simulink model "cp"  (R2012b)
settings: Solver=FixedStepDiscrete  SolverMode=SingleTasking  StartTime=0.0  StopTime=5000  RelTol=1e-3
libraries: shlslibv1 x19
settings Model: synDspstartup=OK  Creator=sszilvasi  LastModifiedBy=sszilvasi
settings DataIOCC: SaveOutput=off  SignalLogging=off  SaveTime=off
settings OptimizationCC: InlineParams=on
settings DebuggingCC: AlgebraicLoopMsg=error  InheritedTsInSrcMsg=none

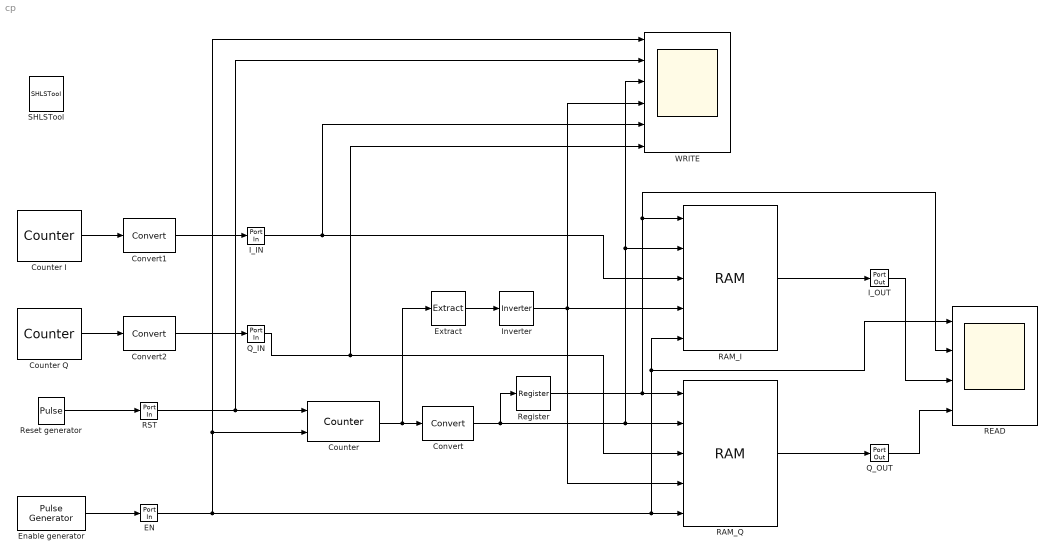
== system cp ==
  Convert : shlslibv1/Signal Operations/Convert  syn_preshift_opr=none  syn_preshift_bits=0  syn_preshift_val=0  syn_out_f=Specify  syn_out_wl=5  syn_out_fl=0  syn_out_dt_sync=unsigned  syn_out_sat=off  syn_out_rnd=Floor (Truncate)  syn_inh_port=off  syn_inh_st=off  syn_inh_stf=1  synBlockType=primitive  synLatency=0  synBlockId=4
  Convert1 : shlslibv1/Signal Operations/Convert  syn_preshift_opr=>>  syn_preshift_bits=9  syn_preshift_val=0  syn_out_f=Specify  syn_out_wl=10  syn_out_fl=9  syn_out_dt_sync=signed  syn_out_sat=off  syn_out_rnd=Floor (Truncate)  syn_inh_port=off  syn_inh_st=off  syn_inh_stf=1  synBlockType=primitive  synLatency=0  synBlockId=4
  Convert2 : shlslibv1/Signal Operations/Convert  syn_preshift_opr=>>  syn_preshift_bits=9  syn_preshift_val=0  syn_out_f=Specify  syn_out_wl=10  syn_out_fl=9  syn_out_dt_sync=signed  syn_out_sat=off  syn_out_rnd=Floor (Truncate)  syn_inh_port=off  syn_inh_st=off  syn_inh_stf=1  synBlockType=primitive  synLatency=0  synBlockId=4
  Counter : shlslibv1/Sources/Counter  syn_rst_port=on  syn_en_port=on  syn_ld_port=off  syn_cnt_type=Up  syn_init_val=0  syn_term_exists=off  syn_rdy_port=off  syn_term_val=127  syn_cnt_f=Specify  syn_cnt_wl=6  syn_cnt_dt=unsigned  syn_cnt_st=-1  synBlockType=primitive  synLatency=0  synBlockId=21
  Counter I : shlslibv1/Sources/Counter  syn_rst_port=off  syn_en_port=off  syn_ld_port=off  syn_cnt_type=Down  syn_init_val=1023  syn_term_exists=off  syn_rdy_port=off  syn_term_val=127  syn_cnt_f=Specify  syn_cnt_wl=10  syn_cnt_dt=unsigned  syn_cnt_st=1  synBlockType=primitive  synLatency=0  synBlockId=21
  Counter Q : shlslibv1/Sources/Counter  syn_rst_port=off  syn_en_port=off  syn_ld_port=off  syn_cnt_type=Up  syn_init_val=0  syn_term_exists=off  syn_rdy_port=off  syn_term_val=127  syn_cnt_f=Specify  syn_cnt_wl=10  syn_cnt_dt=unsigned  syn_cnt_st=1  synBlockType=primitive  synLatency=0  synBlockId=21
  EN : shlslibv1/Ports & Subsystems/Port In  syn_out_wl=1  syn_out_fl=0  syn_out_dt=unsigned  syn_out_st=-1  syn_capture=off  syn_register=on  syn_out_sat=off  syn_out_rnd=on  synBlockType=port  synLatency=1  synBlockId=0
  Enable generator : shlslibv1/Sources/Pulse Generator  syn_siggentype=Step (0 to 1)  syn_usectl=off  syn_trigedge=rising  syn_triginit=low  syn_stpdel=32  syn_impwidth=1  syn_impdel=1  syn_st=1  synBlockType=custom  synLatency=0
  Extract : shlslibv1/Signal Operations/Extract  syn_extract_vec=5  synBlockType=primitive  synLatency=0  synBlockId=17
  I_IN : shlslibv1/Ports & Subsystems/Port In  syn_out_wl=10  syn_out_fl=9  syn_out_dt=signed  syn_out_st=-1  syn_capture=off  syn_register=on  syn_out_sat=off  syn_out_rnd=on  synBlockType=port  synLatency=1  synBlockId=0
  I_OUT : shlslibv1/Ports & Subsystems/Port Out  syn_capture=off  syn_register=on  synBlockType=port  synLatency=1  synBlockId=1
  Inverter : shlslibv1/Math Functions/Inverter  syn_out_f=Automatic  syn_out_wl=16  syn_out_fl=8  syn_out_dt=signed  synBlockType=primitive  synLatency=0  synBlockId=10
  Q_IN : shlslibv1/Ports & Subsystems/Port In  syn_out_wl=10  syn_out_fl=9  syn_out_dt=signed  syn_out_st=-1  syn_capture=off  syn_register=on  syn_out_sat=off  syn_out_rnd=on  synBlockType=port  synLatency=1  synBlockId=0
  Q_OUT : shlslibv1/Ports & Subsystems/Port Out  syn_capture=off  syn_register=on  synBlockType=port  synLatency=1  synBlockId=1
  RAM_I : shlslibv1/Memories/RAM  syn_ram_depth=32  syn_read_nb=1  syn_write_nb=1  syn_rw_nb=0  syn_corereset=off  syn_localreset=off  syn_initial_val=0  syn_enable_port=on  syn_wac=No check  syn_rac=Read-first  synBlockType=primitive  synLatency=1  synBlockId=111
  RAM_Q : shlslibv1/Memories/RAM  syn_ram_depth=32  syn_read_nb=1  syn_write_nb=1  syn_rw_nb=0  syn_corereset=off  syn_localreset=off  syn_initial_val=0  syn_enable_port=on  syn_wac=No check  syn_rac=Read-first  synBlockType=primitive  synLatency=1  synBlockId=111
  READ : Scope  NumInputPorts=4
      settings: YMin=-0~-0~-5~-5  YMax=1024~1024~5~5
  RST : shlslibv1/Ports & Subsystems/Port In  syn_out_wl=1  syn_out_fl=0  syn_out_dt=unsigned  syn_out_st=-1  syn_capture=off  syn_register=on  syn_out_sat=off  syn_out_rnd=on  synBlockType=port  synLatency=1  synBlockId=0
  Register : shlslibv1/Memories/Register  syn_delay_val=1  syn_rst_port=off  syn_en_port=off  synBlockType=custom  synLatency=1
  Reset generator : DiscretePulseGenerator  Period=48  PhaseDelay=32
  SHLSTool : shlslibv1/SHLSTool  synBlockType=tool  syn_dsp_mode=FPGA
  WRITE : Scope  NumInputPorts=6
      settings: YMin=-5~-5~-0~-0~-5~-5  YMax=5~5~64~64~5~5  SaveName=ScopeData3
  wires:
  I_IN/1 -> RAM_I/3, WRITE/5
  Q_IN/1 -> WRITE/6, RAM_Q/3
  RAM_I/1 -> I_OUT/1
  RAM_Q/1 -> Q_OUT/1
  Counter/1 -> Convert/1, Extract/1
  Convert/1 -> Register/1, RAM_Q/2, WRITE/3, RAM_I/2
  EN/1 -> READ/1, RAM_I/5, RAM_Q/5, Counter/2, WRITE/1
  RST/1 -> WRITE/2, Counter/1
  Counter I/1 -> Convert1/1
  Counter Q/1 -> Convert2/1
  Enable generator/1 -> EN/1
  Reset generator/1 -> RST/1
  Convert1/1 -> I_IN/1
  Convert2/1 -> Q_IN/1
  Extract/1 -> Inverter/1
  Inverter/1 -> WRITE/4, RAM_I/4, RAM_Q/4
  I_OUT/1 -> READ/3
  Q_OUT/1 -> READ/4
  Register/1 -> READ/2, RAM_I/1, RAM_Q/1
